simulink model "integracion"  (Simulink 8.5)
settings: Solver=ode4  StartTime=0.0  StopTime=4.0  FixedStep=.001  RelTol=1e-3
settings Model: Creator=ULTIMATE HP  LastModifiedBy=Benjamin Nicolas
settings DebuggingCC: SolverPrmCheckMsg=warning  FcnCallInpInsideContextMsg=UseLocalSettings

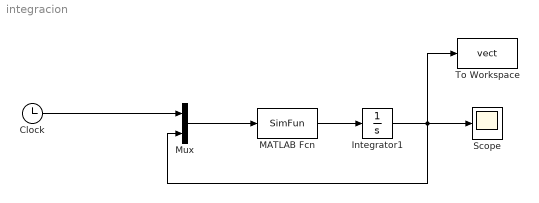
== system integracion ==
  Clock : Clock
  Integrator1 : Integrator  InitialCondition=2
  MATLAB Fcn : MATLABFcn  MATLABFcn=SimFun
  Mux : Mux  Inputs=2
  Scope : Scope
  To Workspace : ToWorkspace  VariableName=vect  SampleTime=-1
  wires:
  MATLAB Fcn/1 -> Integrator1/1
  Integrator1/1 -> Scope/1, Mux/2, To Workspace/1
  Mux/1 -> MATLAB Fcn/1
  Clock/1 -> Mux/1
